simulink model "Copy_of_VehicleFollowing1"  (R2021a)
settings: Solver=VariableStepAuto  StartTime=0.0  StopTime=100  RelTol=1e-3
values from neighbouring files (symbols this model uses):
  acceleration_due_to_gravity = 9.807    [matlab.mat]
libraries: vrlib x3, sim3dautolib x3, simulink x2, mpcadaslib x1, sim3dlib x1
settings Model: Creator=DELL  LastModifiedBy=USER
settings SolverCC: AlgebraicLoopSolver=TrustRegion
settings DataIOCC: ReturnWorkspaceOutputs=off
settings DebuggingCC: SFMachineParentedDataDiag=warning  ArithmeticOperatorsInVariantConditions=warning
settings SFSimCC: CustomCodeUndefinedFunction=UseInterfaceOnly  SimTargetLang=C++

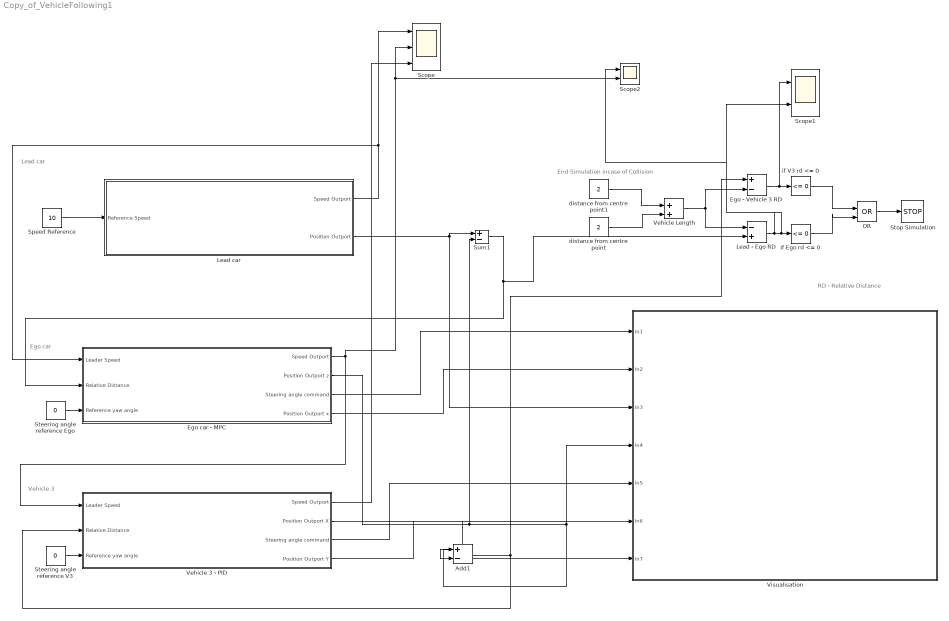
== system Copy_of_VehicleFollowing1 ==
  note: RD - Relative Distance
  note: End Simulation incase of Collision
  note: Ego car
  note: Lead car
  note: Vehicle 3
  Add1 : Sum  Inputs=+-
  Ego - Vehicle 3 RD : Sum  Inputs=+-
  Ego car - MPC : Subsystem  mask{Pos=20, Speed=12}
      mask prompts: Pos "Initial Position"; Speed "Initial Speed"
      mask TypeOptions Pos: Initial Position Z/Value
      mask TypeOptions Speed: Initial Speed/Value
  Lead - Ego RD : Sum  Inputs=-+
  Lead car : Subsystem  mask{Pos=40, Speed=5}
      mask prompts: Pos "Initial Position"; Speed "Initial Speed"
      mask TypeOptions Pos: Initial Position/Value
      mask TypeOptions Speed: Initial Speed/Value
  OR : Logic  Operator=OR  IconShape=distinctive  AllPortsSameDT=off  OutDataTypeStr=boolean
  Scope : Scope  NumInputPorts=3
  Scope1 : Scope  NumInputPorts=2
  Scope2 : Scope  NumInputPorts=2
  Speed Reference : Constant  Value=10
  Steering angle reference Ego : Constant  Value=0
  Steering angle reference V3 : Constant  Value=0
  Stop Simulation : Stop
  Sum1 : Sum  Inputs=|+-
  Vehicle 3 - PID : Subsystem  mask{Pos=0, Speed=8.3}
      mask prompts: Pos "Initial Position"; Speed "Initial Speed"
      mask TypeOptions Pos: Initial Position X/Value
      mask TypeOptions Speed: Initial Speed/Value
  Vehicle Length : Sum  Inputs=+|+
  Visualisation : Subsystem
  distance from centre point : Constant  Value=2
  distance from centre point1 : Constant  Value=2
  if Ego rd <= 0 : simulink/Logic and Bit Operations/Compare To Constant  relop=<=  const=0  OutDataTypeStr=boolean
  if V3 rd <= 0 : simulink/Logic and Bit Operations/Compare To Constant  relop=<=  const=0  OutDataTypeStr=boolean
  wires:
  Lead car/2(Position Outport) -> Visualisation/3(In3), Sum1/1
  Speed Reference/1 -> Lead car/1(Reference Speed)
  Ego car - MPC/1(Speed Outport) -> Vehicle 3 - PID/1(Leader Speed), Scope2/2, Scope/2
  Ego car - MPC/2(Position Outport z) -> Add1/1, Visualisation/4(In4), Sum1/2
  Lead car/1(Speed Outport) -> Scope/1, Ego car - MPC/1(Leader Speed)
  Sum1/1 -> Ego car - MPC/2(Relative Distance), Lead - Ego RD/2
  Steering angle reference Ego/1 -> Ego car - MPC/3(Reference yaw angle)
  distance from centre point/1 -> Vehicle Length/2
  distance from centre point1/1 -> Vehicle Length/1
  Vehicle Length/1 -> Lead - Ego RD/1, Ego - Vehicle 3 RD/2
  Lead - Ego RD/1 -> Scope2/1, Scope1/2, if Ego rd <= 0/1
  Vehicle 3 - PID/2(Position Outport X) -> Add1/2, Visualisation/7(In7)
  OR/1 -> Stop Simulation/1
  Ego - Vehicle 3 RD/1 -> Scope1/1, if V3 rd <= 0/1
  if Ego rd <= 0/1 -> OR/2
  Ego car - MPC/3(Steering angle command) -> Visualisation/1(In1)
  Ego car - MPC/4(Position Outport x) -> Visualisation/2(In2)
  Vehicle 3 - PID/3(Steering angle command) -> Visualisation/5(In5)
  Vehicle 3 - PID/4(Position Outport Y) -> Visualisation/6(In6)
  if V3 rd <= 0/1 -> OR/1
  Add1/1 -> Vehicle 3 - PID/2(Relative Distance), Ego - Vehicle 3 RD/1
  Steering angle reference V3/1 -> Vehicle 3 - PID/3(Reference yaw angle)
  Vehicle 3 - PID/1(Speed Outport) -> Scope/3

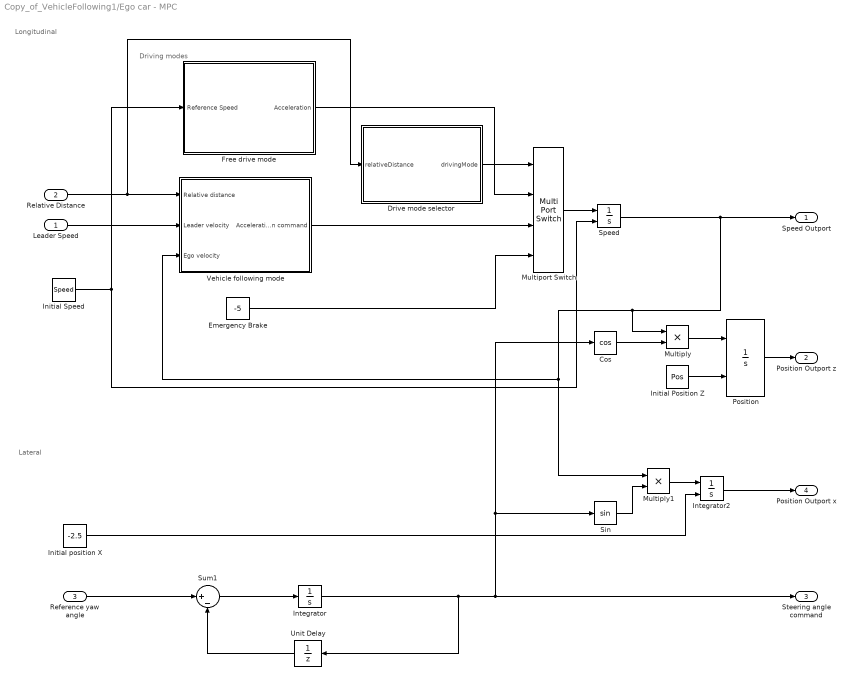
== system Copy_of_VehicleFollowing1/Ego car - MPC ==
  note: Driving modes
  note: Lateral
  note: Longitudinal
  Leader Speed : Inport
  Relative Distance : Inport  Port=2
  Reference yaw angle : Inport  Port=3
  Cos : Trigonometry  Operator=cos
  Drive mode selector : Stateflow chart  TreatAsAtomicUnit=on
  Emergency Brake : Constant  Value=-5
  Free drive mode : Subsystem
  Initial Position Z : Constant  Value=Pos
  Initial Speed : Constant  Value=Speed
  Initial position X : Constant  Value=-2.5
  Integrator : Integrator
  Integrator2 : Integrator  InitialConditionSource=external
  Multiply : Product
  Multiply1 : Product
  Multiport Switch : MultiPortSwitch
  Position : Integrator  InitialConditionSource=external
  Sin : Trigonometry
  Speed : Integrator  InitialConditionSource=external  LimitOutput=on  LowerSaturationLimit=0
  Sum1 : Sum  Inputs=|+-
  Unit Delay : UnitDelay  SampleTime=-1  HasFrameUpgradeWarning=on
  Vehicle following mode : Subsystem
  Speed Outport : Outport  VectorParamsAs1DForOutWhenUnconnected=off
  Position Outport z : Outport  Port=2  VectorParamsAs1DForOutWhenUnconnected=off
  Steering angle command : Outport  Port=3  VectorParamsAs1DForOutWhenUnconnected=off
  Position Outport x : Outport  Port=4  VectorParamsAs1DForOutWhenUnconnected=off
  wires:
  Initial Position Z/1 -> Position/2
  Speed/1 -> Multiply1/1, Vehicle following mode/3(Ego velocity), Multiply/1, Speed Outport/1
  Position/1 -> Position Outport z/1
  Initial Speed/1 -> Free drive mode/1(Reference Speed), Speed/2
  Reference yaw angle/1 -> Sum1/1
  Sum1/1 -> Integrator/1
  Integrator/1 -> Unit Delay/1, Cos/1, Sin/1, Steering angle command/1
  Initial position X/1 -> Integrator2/2
  Cos/1 -> Multiply/2
  Multiply/1 -> Position/1
  Sin/1 -> Multiply1/2
  Multiply1/1 -> Integrator2/1
  Integrator2/1 -> Position Outport x/1
  Unit Delay/1 -> Sum1/2
  Relative Distance/1 -> Drive mode selector/1(relativeDistance), Vehicle following mode/1(Relative distance)
  Leader Speed/1 -> Vehicle following mode/2(Leader velocity)
  Vehicle following mode/1(Acceleration command) -> Multiport Switch/3
  Emergency Brake/1 -> Multiport Switch/4
  Free drive mode/1(Acceleration) -> Multiport Switch/2
  Drive mode selector/1(drivingMode) -> Multiport Switch/1
  Multiport Switch/1 -> Speed/1

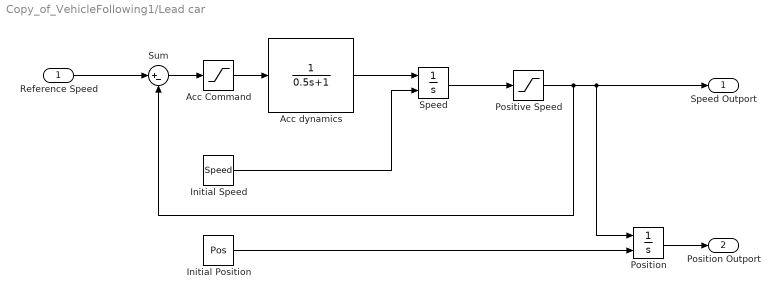
== system Copy_of_VehicleFollowing1/Lead car ==
  Reference Speed : Inport
  Acc Command : Saturate  UpperLimit=2  LowerLimit=-3
  Acc dynamics : TransferFcn  Denominator=[0.5 1]
  Initial Position : Constant  Value=Pos
  Initial Speed : Constant  Value=Speed
  Position : Integrator  InitialConditionSource=external
  Positive Speed : Saturate  UpperLimit=inf  LowerLimit=0
  Speed : Integrator  InitialConditionSource=external
  Sum : Sum  Inputs=|+-
  Speed Outport : Outport  VectorParamsAs1DForOutWhenUnconnected=off
  Position Outport : Outport  Port=2  VectorParamsAs1DForOutWhenUnconnected=off
  wires:
  Initial Speed/1 -> Speed/2
  Acc Command/1 -> Acc dynamics/1
  Speed/1 -> Positive Speed/1
  Sum/1 -> Acc Command/1
  Position/1 -> Position Outport/1
  Acc dynamics/1 -> Speed/1
  Positive Speed/1 -> Sum/2, Speed Outport/1, Position/1
  Initial Position/1 -> Position/2
  Reference Speed/1 -> Sum/1

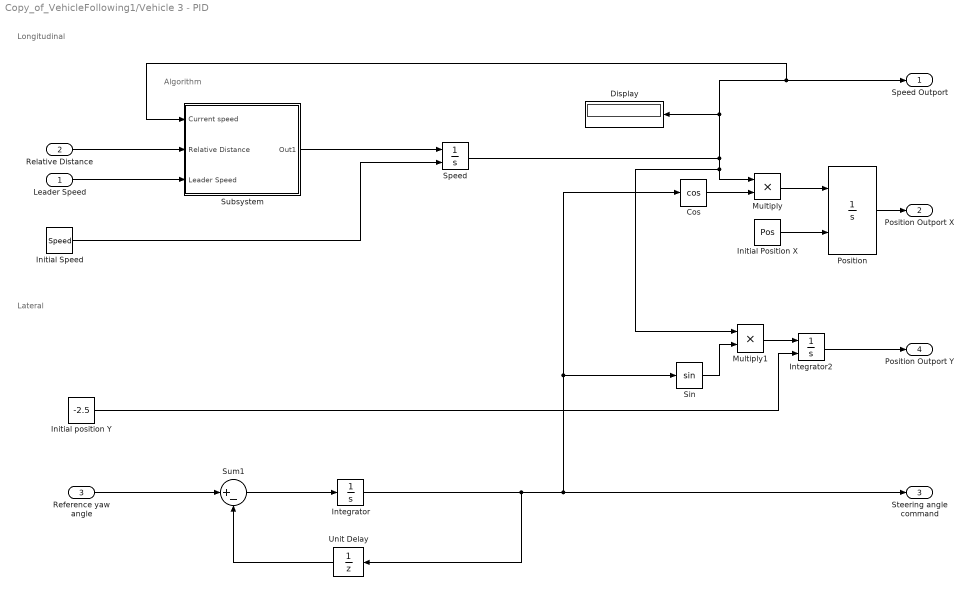
== system Copy_of_VehicleFollowing1/Vehicle 3 - PID ==
  note: Longitudinal
  note: Lateral
  note: Algorithm
  Leader Speed : Inport
  Relative Distance : Inport  Port=2
  Reference yaw angle : Inport  Port=3
  Cos : Trigonometry  Operator=cos
  Display : Display
  Initial Position X : Constant  Value=Pos
  Initial Speed : Constant  Value=Speed
  Initial position Y : Constant  Value=-2.5
  Integrator : Integrator
  Integrator2 : Integrator  InitialConditionSource=external
  Multiply : Product
  Multiply1 : Product
  Position : Integrator  InitialConditionSource=external
  Sin : Trigonometry
  Speed : Integrator  InitialConditionSource=external  LimitOutput=on  LowerSaturationLimit=0
  Subsystem : Subsystem
  Sum1 : Sum  Inputs=|+-
  Unit Delay : UnitDelay  SampleTime=-1  HasFrameUpgradeWarning=on
  Speed Outport : Outport  VectorParamsAs1DForOutWhenUnconnected=off
  Position Outport X : Outport  Port=2  VectorParamsAs1DForOutWhenUnconnected=off
  Steering angle command : Outport  Port=3  VectorParamsAs1DForOutWhenUnconnected=off
  Position Outport Y : Outport  Port=4  VectorParamsAs1DForOutWhenUnconnected=off
  wires:
  Relative Distance/1 -> Subsystem/2(Relative Distance)
  Unit Delay/1 -> Sum1/2
  Integrator2/1 -> Position Outport Y/1
  Multiply1/1 -> Integrator2/1
  Sin/1 -> Multiply1/2
  Multiply/1 -> Position/1
  Cos/1 -> Multiply/2
  Initial position Y/1 -> Integrator2/2
  Integrator/1 -> Steering angle command/1, Sin/1, Cos/1, Unit Delay/1
  Sum1/1 -> Integrator/1
  Reference yaw angle/1 -> Sum1/1
  Initial Speed/1 -> Speed/2
  Position/1 -> Position Outport X/1
  Speed/1 -> Multiply1/1, Multiply/1, Subsystem/1(Current speed), Speed Outport/1, Display/1
  Initial Position X/1 -> Position/2
  Subsystem/1(Out1) -> Speed/1
  Leader Speed/1 -> Subsystem/3(Leader Speed)

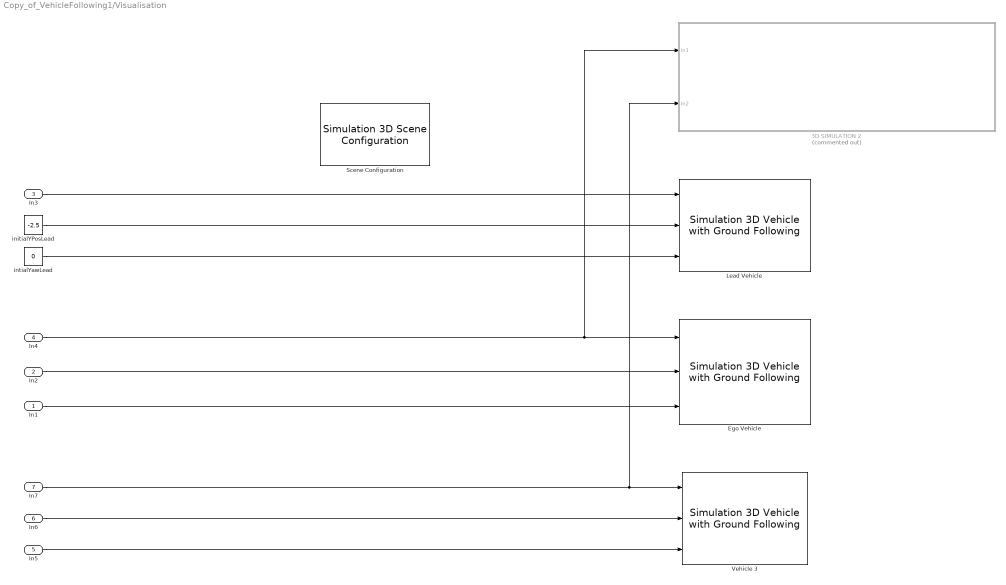
== system Copy_of_VehicleFollowing1/Visualisation ==
  In1 : Inport
  In2 : Inport  Port=2
  In3 : Inport  Port=3
  In4 : Inport  Port=4
  In5 : Inport  Port=5
  In6 : Inport  Port=6
  In7 : Inport  Port=7
  3D SIMULATION 2 : Subsystem  Commented=on
  Ego Vehicle : sim3dautolib/Simulation 3D Vehicle with Ground Following  Priority=-1  PassVehMesh=Sport utility vehicle  MeshPath=/MathWorksSimulation/Vehicles/Muscle/Meshes/SK_MuscleCar.SK_MuscleCar  TrackWidth=1.9  WheelBase=3  WheelRadius=0.35  VehColor=Red  InitialPos=[20, 0, 0]  InitialRot=[0, 0, 0]  ActorName=Ego  SampleTime=0.02  ActorType=SimulinkVehicle  ID=C  aMode=3  ActorTag=Ego  CoordinateScheme=ISO  VehLightsControl=off  HeadlightColor=[ 1, 1, 1 ]  HighBeamIntensity=100000  LowBeamIntensity=60000  HighBeamConeAngle=70  LowBeamConeAngle=70  LeftHeadlightOrientation=[ 0, 0 ]  RightHeadlightOrientation=[ 0, 0 ]  BrakelightIntensity=500  ReverselightIntensity=500  SignallightIntensity=500  SignallightPeriod=1  SignalPulseWidth=50  TransformOutportEnabled=off
      settings: SourceProductBaseCode=DR,UV,VE
  Lead Vehicle : sim3dautolib/Simulation 3D Vehicle with Ground Following  Priority=-1  PassVehMesh=Sedan  MeshPath=/MathWorksSimulation/Vehicles/Muscle/Meshes/SK_MuscleCar.SK_MuscleCar  TrackWidth=1.9  WheelBase=3  WheelRadius=0.35  VehColor=Blue  InitialPos=[40, 0, 0]  InitialRot=[0, 0, 0]  ActorName=Lead Vehicle  SampleTime=0.02  ActorType=SimulinkVehicle  ID=C  aMode=3  ActorTag=Lead Vehicle  CoordinateScheme=ISO  VehLightsControl=off  HeadlightColor=[ 1, 1, 1 ]  HighBeamIntensity=100000  LowBeamIntensity=60000  HighBeamConeAngle=70  LowBeamConeAngle=70  LeftHeadlightOrientation=[ 0, 0 ]  RightHeadlightOrientation=[ 0, 0 ]  BrakelightIntensity=500  ReverselightIntensity=500  SignallightIntensity=500  SignallightPeriod=1  SignalPulseWidth=50  TransformOutportEnabled=off
      settings: SourceProductBaseCode=DR,UV,VE
  Scene Configuration : sim3dlib/Simulation 3D Scene Configuration  Priority=0  ProjectFormat=Default Scenes  SceneDesc=Double lane change  ProjectName=C:\Program Files\MATLAB\R2021a\toolbox\shared\sim3d_projects\automotive_project\UE4\WindowsNoEditor\VehicleSimulation.exe  ScenePath=/Game/Maps/HwStrght  vehTagList={'Ego';'Lead Vehicle';'Scene Origin';'Vehicle 3'}  vehTag=Vehicle 3  OpVisEn=off  Ts=0.02  EnableWindow=on  EnableWeather=off  SunAltitude=40.0  SunAzimuth=90  clouds=10  wind=1  fog=0  rain=0  sensorTag=MainCamera1  sensorId=1  sensorName=MainCamera1  mountLoc=Origin  offsetFlag=off  tmountOffset=[0, 0, 0]  rmountOffset=[0, 0, 0]  HorizontalResolution=1280  VerticalResolution=720  HorizontalFOV=60  mountPoint=[0 0 0]  mountOrientation=[0 0 0]  aMode=3  ID=1
      settings: SourceProductBaseCode=DR,UV,VE
  Vehicle 3 : sim3dautolib/Simulation 3D Vehicle with Ground Following  Priority=-1  PassVehMesh=Muscle car  MeshPath=/MathWorksSimulation/Vehicles/Muscle/Meshes/SK_MuscleCar.SK_MuscleCar  TrackWidth=1.9  WheelBase=3  WheelRadius=0.35  VehColor=White  InitialPos=[0, 0, 0]  InitialRot=[0, 0, 0]  ActorName=Vehicle 3  SampleTime=0.02  ActorType=SimulinkVehicle  ID=C  aMode=3  ActorTag=Vehicle 3  CoordinateScheme=ISO  VehLightsControl=off  HeadlightColor=[ 1, 1, 1 ]  HighBeamIntensity=100000  LowBeamIntensity=60000  HighBeamConeAngle=70  LowBeamConeAngle=70  LeftHeadlightOrientation=[ 0, 0 ]  RightHeadlightOrientation=[ 0, 0 ]  BrakelightIntensity=500  ReverselightIntensity=500  SignallightIntensity=500  SignallightPeriod=1  SignalPulseWidth=50  TransformOutportEnabled=off
      settings: SourceProductBaseCode=DR,UV,VE
  initialYPosLead : Constant  Value=-2.5
  intialYawLead : Constant  Value=0
  wires:
  In2/1 -> Ego Vehicle/2
  In3/1 -> Lead Vehicle/1
  In7/1 -> 3D SIMULATION 2/2(In2), Vehicle 3/1
  In5/1 -> Vehicle 3/3
  In4/1 -> 3D SIMULATION 2/1(In1), Ego Vehicle/1
  In6/1 -> Vehicle 3/2
  initialYPosLead/1 -> Lead Vehicle/2
  intialYawLead/1 -> Lead Vehicle/3
  In1/1 -> Ego Vehicle/3

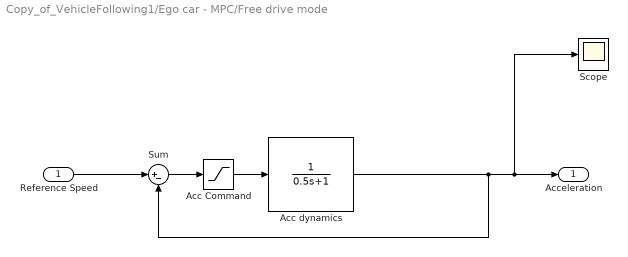
== system Copy_of_VehicleFollowing1/Ego car - MPC/Free drive mode ==
  Reference Speed : Inport
  Acc Command : Saturate  UpperLimit=3  LowerLimit=-3
  Acc dynamics : TransferFcn  Denominator=[0.5 1]
  Scope : Scope
  Sum : Sum  Inputs=|+-
  Acceleration : Outport  VectorParamsAs1DForOutWhenUnconnected=off
  wires:
  Reference Speed/1 -> Sum/1
  Acc Command/1 -> Acc dynamics/1
  Sum/1 -> Acc Command/1
  Acc dynamics/1 -> Sum/2, Scope/1, Acceleration/1

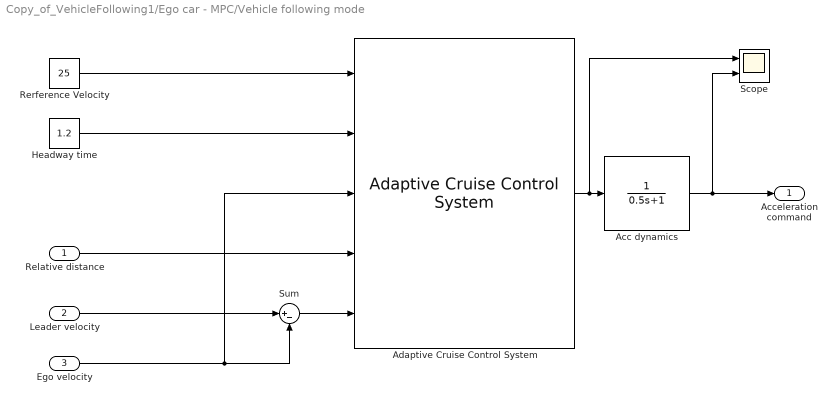
== system Copy_of_VehicleFollowing1/Ego car - MPC/Vehicle following mode ==
  Relative distance : Inport
  Leader velocity : Inport  Port=2
  Ego velocity : Inport  Port=3
  Acc dynamics : TransferFcn  Denominator=[0.5 1]
  Adaptive Cruise Control System : mpcadaslib/Adaptive Cruise Control System  EgoModel=tf(1,[0.5,1,0])  InitialEgoVelocity=25  DefaultSpacing=5  MaxVelocity=14  MinAcceleration=-3  amin_ext=off  MaxAcceleration=2  amax_ext=off  Ts=0.1  PredictionHorizon=200  ControllerBehavior=0.600  suboptimal=off  maxiter=100  datatypeopt=double  optmode=off  trackmode=off
  Headway time : Constant  Value=1.2
  Rerference Velocity : Constant  Value=25
  Scope : Scope  NumInputPorts=2
  Sum : Sum  Inputs=|+-
  Acceleration command : Outport  VectorParamsAs1DForOutWhenUnconnected=off
  wires:
  Ego velocity/1 -> Adaptive Cruise Control System/3, Sum/2
  Headway time/1 -> Adaptive Cruise Control System/2
  Sum/1 -> Adaptive Cruise Control System/5
  Rerference Velocity/1 -> Adaptive Cruise Control System/1
  Relative distance/1 -> Adaptive Cruise Control System/4
  Leader velocity/1 -> Sum/1
  Acc dynamics/1 -> Scope/2, Acceleration command/1
  Adaptive Cruise Control System/1 -> Scope/1, Acc dynamics/1

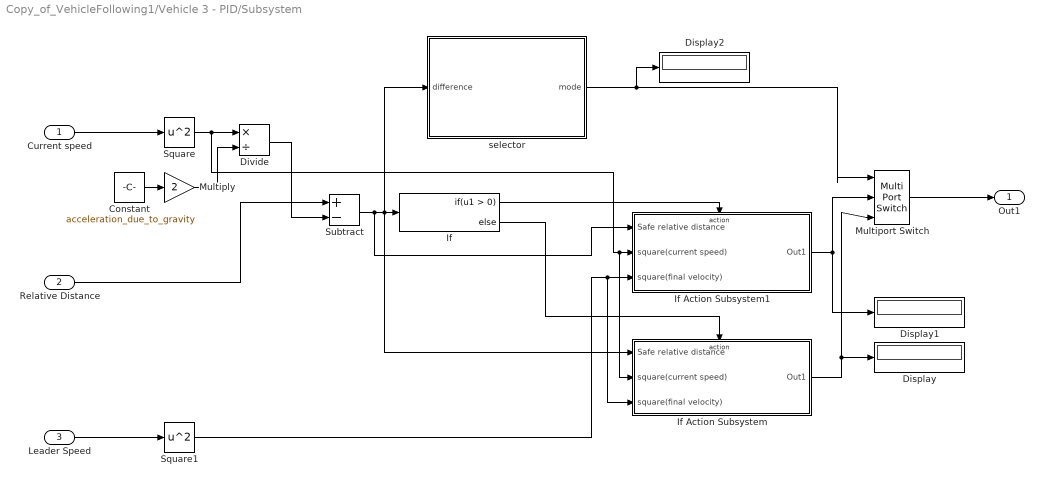
== system Copy_of_VehicleFollowing1/Vehicle 3 - PID/Subsystem ==
  Current speed : Inport
  Relative Distance : Inport  Port=2
  Leader Speed : Inport  Port=3
  Constant : Constant  Value=acceleration_due_to_gravity
  Display : Display
  Display1 : Display
  Display2 : Display
  Divide : Product  Inputs=*/
  If : If
  If Action Subsystem : Subsystem  TreatAsAtomicUnit=on
  If Action Subsystem1 : Subsystem  TreatAsAtomicUnit=on
  Multiply : Gain  Gain=2
  Multiport Switch : MultiPortSwitch  Inputs=2
  Square : Math  Operator=square  SaturateOnIntegerOverflow=on
  Square1 : Math  Operator=square  SaturateOnIntegerOverflow=on
  Subtract : Sum  Inputs=+-
  selector : Stateflow chart  TreatAsAtomicUnit=on
  Out1 : Outport
  wires:
  Square/1 -> If Action Subsystem/2(square(current speed)), If Action Subsystem1/2(square(current speed)), Divide/1
  Constant/1 -> Multiply/1
  Multiply/1 -> Divide/2
  Relative Distance/1 -> Subtract/1
  Divide/1 -> Subtract/2
  Subtract/1 -> If Action Subsystem1/1(Safe relative distance), selector/1(difference), If/1, If Action Subsystem/1(Safe relative distance)
  If/2 -> If Action Subsystem/Action
  If/1 -> If Action Subsystem1/Action
  Leader Speed/1 -> Square1/1
  Square1/1 -> If Action Subsystem/3(square(final velocity)), If Action Subsystem1/3(square(final velocity))
  Current speed/1 -> Square/1
  If Action Subsystem/1(Out1) -> Display/1, Multiport Switch/3
  selector/1(mode) -> Display2/1, Multiport Switch/1
  If Action Subsystem1/1(Out1) -> Multiport Switch/2, Display1/1
  Multiport Switch/1 -> Out1/1

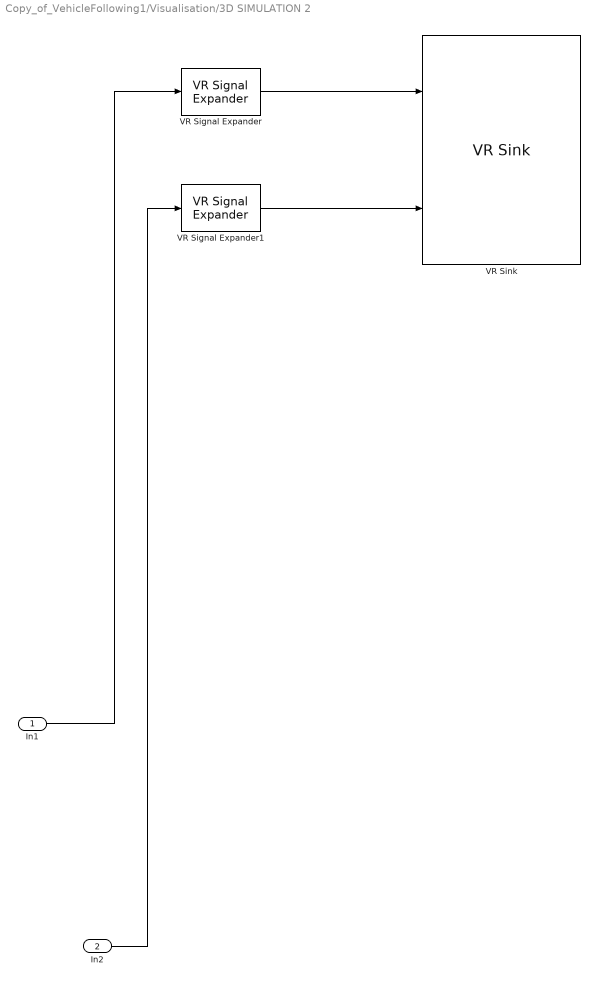
== system Copy_of_VehicleFollowing1/Visualisation/3D SIMULATION 2 ==
  In1 : Inport
  In2 : Inport  Port=2
  VR Signal Expander : vrlib/VR Signal Expander  outwidth=3  outidx=[3]
  VR Signal Expander1 : vrlib/VR Signal Expander  outwidth=3  outidx=[3]
  VR Sink : vrlib/VR Sink  InstantiateOnLoad=on  SampleTime=0.02  ViewEnable=on  RemoteChange=off  RemoteView=off  FieldsWritten=Car_Red.translation.3.1.1.double#Car_Blue.translation.3.1.1.double  WorldFileName=res\PlatoonWorld.WRL  AutoView=off  VideoDimensions=[]  AllowVariableSize=off
  wires:
  In2/1 -> VR Signal Expander1/1
  VR Signal Expander1/1 -> VR Sink/2
  VR Signal Expander/1 -> VR Sink/1
  In1/1 -> VR Signal Expander/1

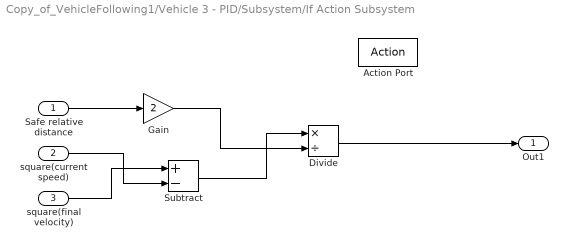
== system Copy_of_VehicleFollowing1/Vehicle 3 - PID/Subsystem/If Action Subsystem ==
  Safe relative distance : Inport
  square(current speed) : Inport  Port=2
  square(final velocity) : Inport  Port=3
  Action Port : ActionPort  ActionPortLabel=else
  Divide : Product  Inputs=*/
  Gain : Gain  Gain=2
  Subtract : Sum  Inputs=+-
  Out1 : Outport
  wires:
  Subtract/1 -> Divide/1
  Divide/1 -> Out1/1
  Safe relative distance/1 -> Gain/1
  square(final velocity)/1 -> Subtract/1
  square(current speed)/1 -> Subtract/2
  Gain/1 -> Divide/2

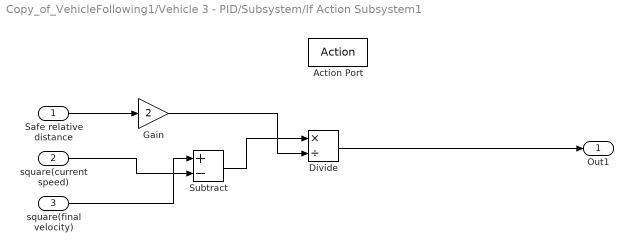
== system Copy_of_VehicleFollowing1/Vehicle 3 - PID/Subsystem/If Action Subsystem1 ==
  Safe relative distance : Inport
  square(current speed) : Inport  Port=2
  square(final velocity) : Inport  Port=3
  Action Port : ActionPort  ActionPortLabel=if(u1 > 0)
  Divide : Product  Inputs=*/
  Gain : Gain  Gain=2
  Subtract : Sum  Inputs=+-
  Out1 : Outport
  wires:
  Subtract/1 -> Divide/1
  Divide/1 -> Out1/1
  square(final velocity)/1 -> Subtract/1
  square(current speed)/1 -> Subtract/2
  Safe relative distance/1 -> Gain/1
  Gain/1 -> Divide/2

== stateflow chart Copy_of_VehicleFollowing1/Vehicle 3 - PID/Subsystem/selector ==
  state positive
    entry:
    mode = 1;
  state negative
    entry:
    mode = 2;
  (default) -> positive
  negative -> positive : [difference > 0]
  positive -> negative : [difference <= 0]
  data: difference input; mode output

== stateflow chart Copy_of_VehicleFollowing1/Ego car - MPC/Drive mode selector ==
  state FreeDrive
    entry:
    drivingMode = 1;
  state VehicleFollowing
    entry:
    drivingMode = 2;
  state EmergencyBrake
    entry:
    drivingMode = 3;
  (default) -> FreeDrive
  VehicleFollowing -> FreeDrive [order 1] : [relativeDistance > 25]
  FreeDrive -> VehicleFollowing [order 1] : [relativeDistance <= 25]
  FreeDrive -> EmergencyBrake [order 2] : [relativeDistance <= 10]
  VehicleFollowing -> EmergencyBrake [order 2] : [relativeDistance <= 10]
  EmergencyBrake -> VehicleFollowing : [relativeDistance >10]
  data: relativeDistance input; drivingMode output
